simulink model "FSK_with_cos"  (R2015a)
settings: Solver=ode45  StartTime=0.0  StopTime=10.0  RelTol=1e-3
libraries: commdigbbndfm2 x2, commfilt2 x2, commchan3 x1, commsink2 x1, commrandsrc2 x1
settings Model: Creator=Yasmeen  LastModifiedBy=Yasmeen

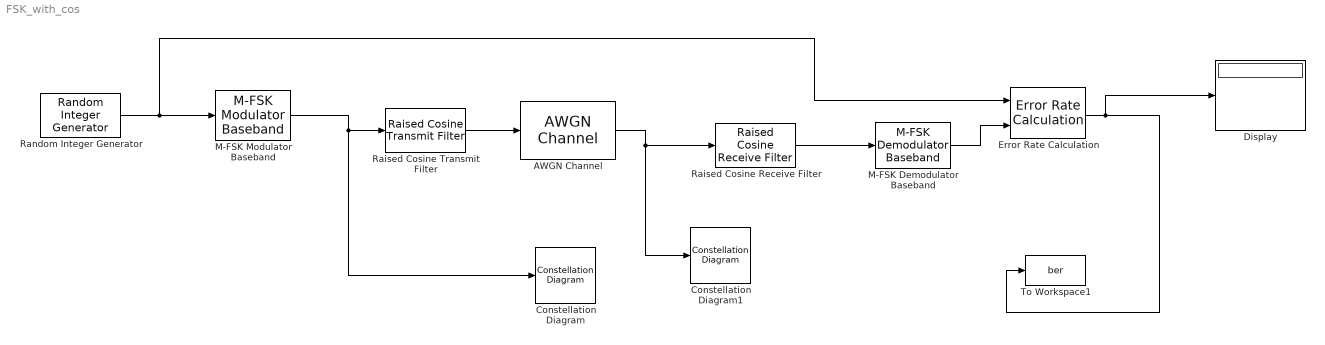
== system FSK_with_cos ==
  AWGN Channel : commchan3/AWGN Channel  InputProcessing=Columns as channels (frame based)  seed=67  noiseMode="Signal to noise ratio  (Eb/No)"  EbNodB=EbNo  EsNodB=10  SNRdB=10  bitsPerSym=3  Ps=1  Tsym=1  variance=1
  Constellation Diagram : ConstellationDiagram
  Constellation Diagram1 : ConstellationDiagram
  Display : Display
  Error Rate Calculation : commsink2/Error Rate Calculation  N=10  st_delay=0  cp_mode=Entire frame  subframe=[]  PMode=Port  WsName=ErrorVec  RsMode2=off  stop=off  numErr=100  maxBits=1e6
  M-FSK Demodulator Baseband : commdigbbndfm2/M-FSK Demodulator Baseband  M=8  OutType=Integer  Dec=Gray  freqSep=6  numSamp=17  RateOptions=Enforce single-rate processing  outDataType=double
  M-FSK Modulator Baseband : commdigbbndfm2/M-FSK Modulator Baseband  M=8  InType=Integer  Enc=Gray  freqSep=6  phaseType=Continuous  numSamp=17  RateOptions=Enforce single-rate processing  outDataType=double
  Raised Cosine Receive Filter : commfilt2/Raised Cosine Receive Filter  filtType=Normal  N=8  filtSpan=10  currentFiltSpan=10  D=5  R=0.2  sampMode=Mute  saveAsFlag=0  rateMode=Downsampling  downFactor=8  downOffset=0  framing=Enforce single-rate processing  InputProcessing=Columns as channels (frame based)  checkGain=Normalized  filterGain=1  checkCoeff=off  variableName=rcRxFilt  launchFVT=on  roundingMode=Floor  overflowMode=off
  Raised Cosine Transmit Filter : commfilt2/Raised Cosine Transmit Filter  filtType=Normal  filtSpan=10  currentFiltSpan=10  D=5  R=0.2  sampMode=Mute  saveAsFlag=0  N=8  framing=Enforce single-rate processing  InputProcessing=Columns as channels (frame based)  checkGain=Normalized  filterGain=1  checkCoeff=off  variableName=rcTxFilt  launchFVT=on  roundingMode=Floor  overflowMode=off
  Random Integer Generator : commrandsrc2/Random Integer Generator  mul=8  seed=37  Ts=1  frameBased=on  sampPerFrame=100  orient=off  outDataType=double
  To Workspace1 : ToWorkspace  VariableName=ber  SampleTime=-1
      settings: MaxDataPoints=2  Save2DSignal=2-D array (concatenate along first dimension)
  wires:
  M-FSK Modulator Baseband/1 -> Constellation Diagram/1, Raised Cosine Transmit Filter/1
  AWGN Channel/1 -> Constellation Diagram1/1, Raised Cosine Receive Filter/1
  M-FSK Demodulator Baseband/1 -> Error Rate Calculation/2
  Error Rate Calculation/1 -> To Workspace1/1, Display/1
  Random Integer Generator/1 -> M-FSK Modulator Baseband/1, Error Rate Calculation/1
  Raised Cosine Receive Filter/1 -> M-FSK Demodulator Baseband/1
  Raised Cosine Transmit Filter/1 -> AWGN Channel/1
